simulink model "open_loop_ctrl"  (R2018a)
settings: Solver=VariableStepAuto  StartTime=0.0  StopTime=10.0  RelTol=1e-3
undefined symbols (not defined in the file or in its folder): p
settings Model: Creator=mz-171742  LastModifiedBy=mz-171742

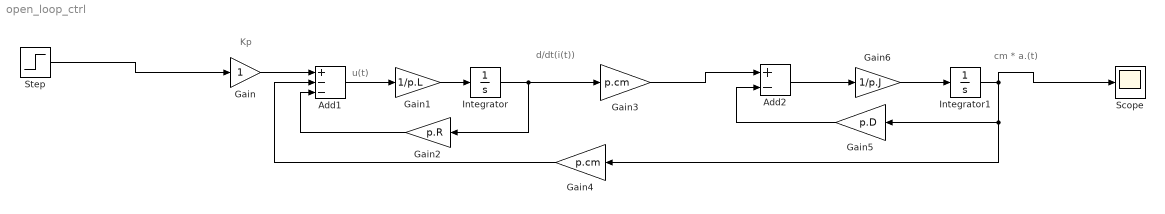
== system open_loop_ctrl ==
  note: Kp
  note: u(t)
  note: cm * a.(t)
  note: d/dt(i(t))
  Add1 : Sum  Inputs=+--
  Add2 : Sum  Inputs=+-
  Gain : Gain
  Gain1 : Gain  Gain=1/p.L
  Gain2 : Gain  Gain=p.R
  Gain3 : Gain  Gain=p.cm
  Gain4 : Gain  Gain=p.cm
  Gain5 : Gain  Gain=p.D
  Gain6 : Gain  Gain=1/p.J
  Integrator : Integrator
  Integrator1 : Integrator
  Scope : Scope
  Step : Step  Time=0  SampleTime=0
  wires:
  Gain1/1 -> Integrator/1
  Gain3/1 -> Add2/1
  Add2/1 -> Gain6/1
  Gain6/1 -> Integrator1/1
  Gain4/1 -> Add1/2
  Add1/1 -> Gain1/1
  Integrator/1 -> Gain2/1, Gain3/1
  Integrator1/1 -> Scope/1, Gain4/1, Gain5/1
  Gain5/1 -> Add2/2
  Gain/1 -> Add1/1
  Gain2/1 -> Add1/3
  Step/1 -> Gain/1
